simulink model "passive_susp"  (R2019a)
settings: Solver=VariableStepAuto  StartTime=0.0  StopTime=2  RelTol=1e-3
values from neighbouring files (symbols this model uses):
  Cs = 1779.8    [suspension.m]
  Cus = 1592    [suspension.m]
  Ks = 22000    [suspension.m]
  Kus = 176000    [suspension.m]
  Ms = 400    [suspension.m]
  Mus = 40    [suspension.m]
settings Model: Creator=Aly  LastModifiedBy=Aly

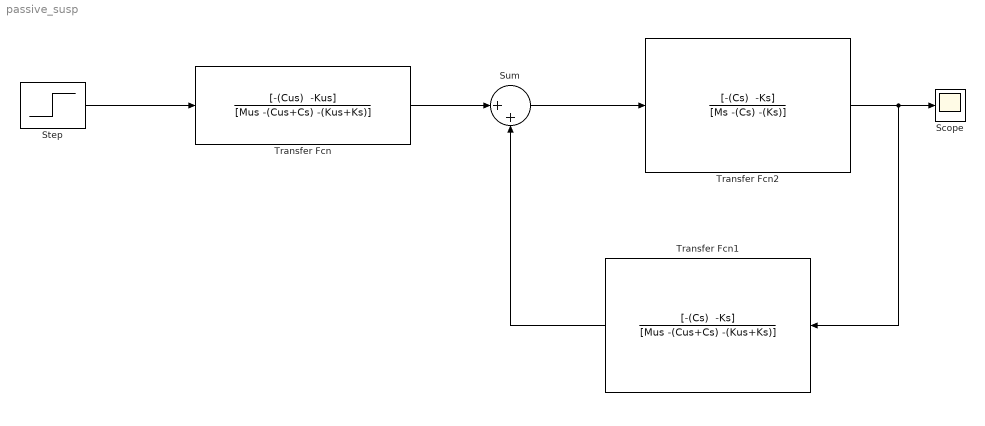
== system passive_susp ==
  Scope : Scope
  Step : Step  SampleTime=0
  Sum : Sum  Inputs=|++
  Transfer Fcn : TransferFcn  Numerator="[-(Cus)  -Kus]"  Denominator=[Mus -(Cus+Cs) -(Kus+Ks)]
  Transfer Fcn1 : TransferFcn  Numerator="[-(Cs)  -Ks]"  Denominator=[Mus -(Cus+Cs) -(Kus+Ks)]
  Transfer Fcn2 : TransferFcn  Numerator="[-(Cs)  -Ks]"  Denominator=[Ms -(Cs) -(Ks)]
  wires:
  Step/1 -> Transfer Fcn/1
  Transfer Fcn1/1 -> Sum/2
  Transfer Fcn/1 -> Sum/1
  Sum/1 -> Transfer Fcn2/1
  Transfer Fcn2/1 -> Transfer Fcn1/1, Scope/1
